simulink model "in_valve"  (R2024a)
settings: Solver=VariableStepAuto  StartTime=0.0  StopTime=10.0  RelTol=1e-3
settings Model: Creator=pc  LastModifiedBy=pc

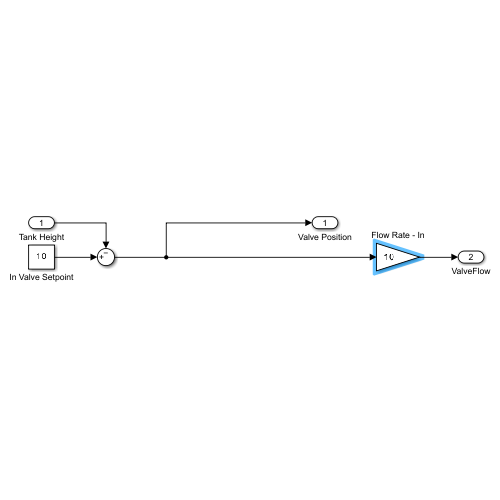
[thumbnail: Simulink's stored preview of the top-level diagram]
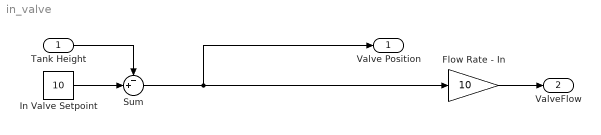
== system in_valve ==
  Tank Height : Inport
  Flow Rate - In : Gain  Gain=10  OutDataTypeStr=Inherit: Inherit via back propagation  SaturateOnIntegerOverflow=on  ParamDataTypeStr=Inherit: Same as input
  In Valve Setpoint : Constant  Value=10
  Sum : Sum  Inputs=-+|
  Valve Position : Outport  InitialOutput=0  VectorParamsAs1DForOutWhenUnconnected=off
  ValveFlow : Outport  Port=2  InitialOutput=0  VectorParamsAs1DForOutWhenUnconnected=off
  wires:
  Sum/1 -> Flow Rate - In/1, Valve Position/1
  Tank Height/1 -> Sum/1
  Flow Rate - In/1 -> ValveFlow/1
  In Valve Setpoint/1 -> Sum/2
